simulink model "FullSystem"  (R2025a)
settings: Solver=VariableStepAuto  StartTime=0.0  StopTime=5  MaxStep=0.00001  RelTol=1e-3
libraries: fl_lib x11, nesl_utility x4, ee_lib x1
settings Model: Creator=yaremadzulynsky  LastModifiedBy=yaremadzulynsky

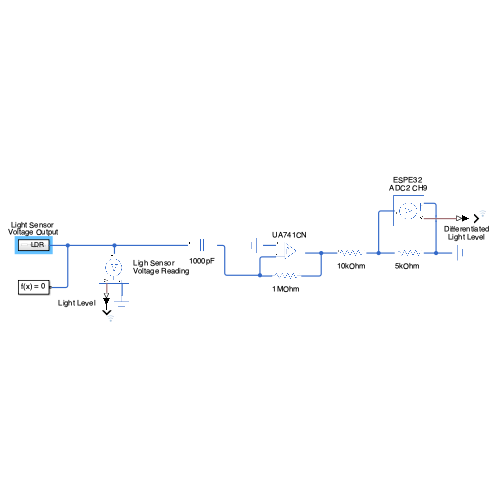
[thumbnail: Simulink's stored preview of the top-level diagram]
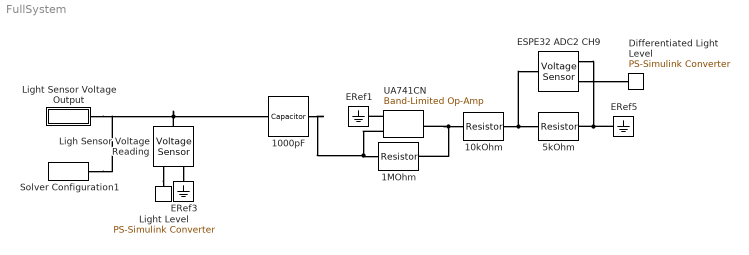
== system FullSystem ==
  1000pF : fl_lib/Electrical/Electrical Elements/Capacitor  c=0.1 uF  r=1e-6 Ohm  g=0 1/Ohm  i_specify=off  i_priority=None  i=0 A  i_nominal_specify=off  i_nominal_value=1  i_nominal_unit=A  v_specify=off  v_priority=None  v=0 V  v_nominal_specify=off  v_nominal_value=1  v_nominal_unit=V  vc_specify=off  vc_priority=High  vc=0 V  vc_nominal_specify=off  vc_nominal_value=1  vc_nominal_unit=V
  10kOhm : fl_lib/Electrical/Electrical Elements/Resistor  R=10 kOhm  i_specify=off  i_priority=None  i=0 A  i_nominal_specify=off  i_nominal_value=1  i_nominal_unit=A  v_specify=off  v_priority=None  v=0 V  v_nominal_specify=off  v_nominal_value=1  v_nominal_unit=V
  1MOhm : fl_lib/Electrical/Electrical Elements/Resistor  R=1 MOhm  i_specify=off  i_priority=None  i=0 A  i_nominal_specify=off  i_nominal_value=1  i_nominal_unit=A  v_specify=off  v_priority=None  v=0 V  v_nominal_specify=off  v_nominal_value=1  v_nominal_unit=V
  "5kOhm " : fl_lib/Electrical/Electrical Elements/Resistor  R=5 kOhm  i_specify=off  i_priority=None  i=0 A  i_nominal_specify=off  i_nominal_value=1  i_nominal_unit=A  v_specify=off  v_priority=None  v=0 V  v_nominal_specify=off  v_nominal_value=1  v_nominal_unit=V
  "Differentiated Light Level " : nesl_utility/PS-Simulink Converter  PhysicalDomain=network_engine_domain  SubClassName=ps_output  LeftPortType=input  RightPortType=output  PseudoPeriodic=off  Frequencies=[]  VectorFormat=inherit  Unit=inherit  AffineConversion=off
  ERef1 : fl_lib/Electrical/Electrical Elements/Electrical Reference
  ERef3 : fl_lib/Electrical/Electrical Elements/Electrical Reference
  ERef5 : fl_lib/Electrical/Electrical Elements/Electrical Reference
  ESPE32 ADC2 CH9 : fl_lib/Electrical/Electrical Sensors/Voltage Sensor
  Ligh Sensor Voltage Reading : fl_lib/Electrical/Electrical Sensors/Voltage Sensor
  Light Level : nesl_utility/PS-Simulink Converter  PhysicalDomain=network_engine_domain  SubClassName=ps_output  LeftPortType=input  RightPortType=output  PseudoPeriodic=off  Frequencies=[]  VectorFormat=inherit  Unit=inherit  AffineConversion=off
  Light Sensor Voltage Output : Subsystem
  Solver Configuration1 : nesl_utility/Solver Configuration  PhysicalDomain=network_engine_domain  SubClassName=solver  LeftPortType=input  RightPortType=generic  Tones=[]  Harmonics=[]  SimulateNoise=off  Profile=off  UseLocalSampling=off  EnableSwitchedLinearOptims=on  FrequencyDomain=off  UseCCode=off  RelTol=0.001  AbsTol=0.001  MinStep=1e-09  ToWorkspace=off  RevertToSquareIcSolve=off  NumHomotopyIterations=100  PhasorMode=off  PhasorModeNumHarmonics=1  ConsistencySolver=NEWTON_XTOL_AFTER_FTOL  IndexReductionMethod=DerivativeReplacement  DoDC=off  ResidualTolerance=1e-09  ConsistencyTolSource=GLOBAL  ConsistencyAbsTol=0.001  ConsistencyRelTol=0.001  ConsistencyTolFactor=0.001  UseLocalSolver=off  LocalSolverChoice=NE_BACKWARD_EULER_ADVANCER  ResolveIndetEquations=on  FunctionEvalNumThread=1  LocalSolverSampleTime=0.001  DoFixedCost=off  MaxNonlinIter=3  MaxModeIter=2  ComputeImpulses=off  ImpulseIterations=2  LinearAlgebra=auto  LinearAlgebraNumThread=0  EquationFormulation=NE_TIME_EF  DelaysMemoryBudget=1024  AutomaticFiltering=on  FilteringTimeConstant=0.001  PartitionStorageMethod=AS_NEEDED  PartitionMemoryBudget=1024  PartitionMethod=ROBUST  MultibodyUseLocalSolver=off  MultibodyLocalSolverChoice=ODE1  MultibodyLocalSolverSampleTime=0.001
  UA741CN : ee_lib/Integrated Circuits/Band-Limited Op-Amp  A=1000  Rin=2e6 Ohm  Rout=75 Ohm  Vmin=0 V  Vmax=5 V  Vdotmax=500000 V/s  f=1e6 Hz  V0=0 V
  connections:
  10kOhm/LConn1 -- UA741CN/RConn1 -- 1MOhm/RConn1
  Ligh Sensor Voltage Reading/LConn1 -- Light Sensor Voltage Output/LConn1 -- Solver Configuration1/RConn1 -- 1000pF/LConn1
  10kOhm/RConn1 -- ESPE32 ADC2 CH9/LConn1 -- "5kOhm "/LConn1
  ERef5/LConn1 -- ESPE32 ADC2 CH9/RConn2 -- "5kOhm "/RConn1
  Ligh Sensor Voltage Reading/RConn2 -- ERef3/LConn1
  Ligh Sensor Voltage Reading/RConn1 -- Light Level/LConn1
  ESPE32 ADC2 CH9/RConn1 -- "Differentiated Light Level "/LConn1
  1000pF/RConn1 -- UA741CN/LConn2 -- 1MOhm/LConn1
  UA741CN/LConn1 -- ERef1/LConn1

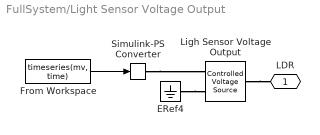
== system FullSystem/Light Sensor Voltage Output ==
  ERef4 : fl_lib/Electrical/Electrical Elements/Electrical Reference
  From Workspace : FromWorkspace  VariableName=timeseries(mv, time)
  Ligh Sensor Voltage Output : fl_lib/Electrical/Electrical Sources/Controlled Voltage Source
  Simulink-PS Converter : nesl_utility/Simulink-PS Converter  PhysicalDomain=network_engine_domain  SubClassName=ps_input  LeftPortType=input  RightPortType=output  PseudoPeriodic=off  Frequencies=[]  NoiseDistribution=none  NoiseParameters=[]  Unit=1  AffineConversion=off  FilteringAndDerivatives=provide  SimscapeFilterOrder=1  InputFilterTimeConstant=0.001  UdotUserProvided=0
  "LDR " : PMIOPort  Side=Left
  wires:
  From Workspace/1 -> Simulink-PS Converter/1
  connections:
  Ligh Sensor Voltage Output/LConn1 -- "LDR "/RConn1
  Simulink-PS Converter/RConn1 -- Ligh Sensor Voltage Output/RConn1
  ERef4/LConn1 -- Ligh Sensor Voltage Output/RConn2
